simulink subsystem "PvtSubSys_HMI"  (R2020b)
settings: Solver=VariableStepAuto  StartTime=0.0  StopTime=10.0  RelTol=1e-3
undefined symbols (not defined in the file): P_HMI_LDW_LKAWarnTime, P_HMI_ObjectTypeFilter, P_HMI_WarnFormLDWReq
libraries: simulink x212, TrueDurationTime x6
(part 4 of 8)

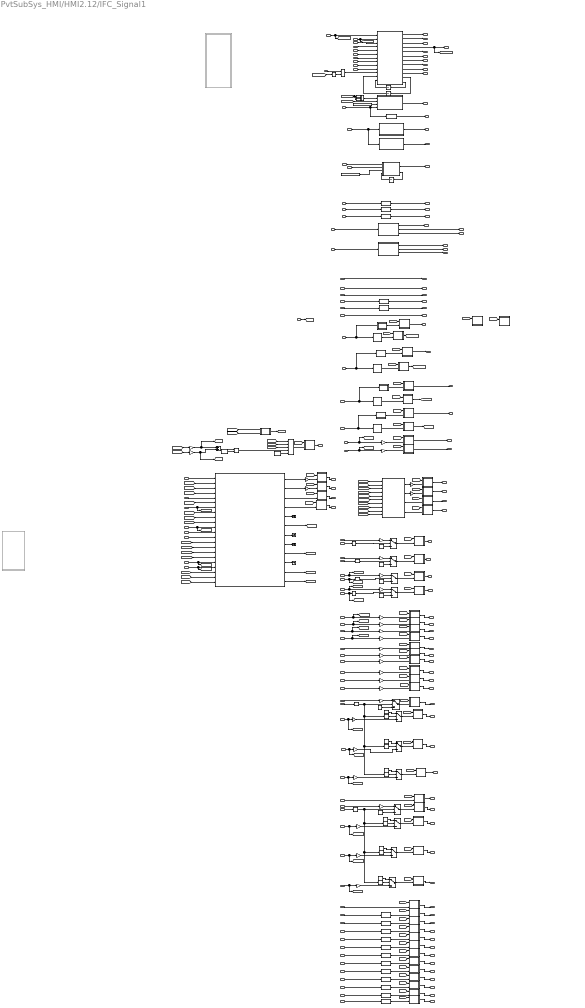
== system PvtSubSys_HMI/HMI2.12/IFC_Signal1 ==
  note: 按照开关请求
      | （ESS_PedSwtReq/ESS_VehSwtReq）
      | 进行正常值发送
  note: 需要添加 标定值
  note: 车道类型：目前只能显示车道线，还无法
      | 显示车道边界
  note: ELK 关联 3L功能 存在漏洞 2020/12/02
      |
      | 无故障：  0x0：No error
      | IFC故障： 0x2:LKA error
      | IFC无故障，RSDS故障：0x4:ELK error
      | error优先级：ELK>3L
      | （2）目前LKAResp 输出存在问题；无法与开关关联
      | 目前功能优先级；
      | TJA>ELK>3L
  note: 1.3.5——>1 solid
      | 2.4.6——>1 Dashed
      | 10.12.13——>1 Rode Edge
      | 8——>减速线（非虚线）
      | 14——>减速线（虚线）
  note: TJA_Off(0)
      |        TJA_Idle(1)
      |        TJA_Ready(2)
      |        TJA_Active(3)
      |        TJA_Error(7)
      |        TJA_SafeStop(9)
  note: Fusion:LaneAvailability
  note: Fusion:CameraBlockageSts
  note: Fusion:IFCCalibrationSts
  note: 0x0=UNDECIDED |
      | 0x1=SOLID |
      | 0x2=DASHED |
      | 0x3=DOUBLE_SOLID_DASHED |
      | 0x4=DOUBLE_DASHED_SOLID |
      | 0x5=DOUBLE_SOLID_SOLID |
      | 0x6=DOUBLE_DASHED_DASHED |
      | 0x7=BOTTS |
      | 0x8=DECELERATION |
      | 0x9=HOV_LANE |
      | 0xA=ROAD_EDGE |
      | 0xB=ELEVATED_STRUCTURE |
      | 0xC=LCURB |
      | 0xD=CONES_POLES |
      | 0xE=PARKED_CARS
  note: 0x0:Inactive
      | 0x1:Left Active
      | 0x2:Right active
      | 0x3:Reserved
  note: 0x0:Inactive
      | 0x1:Left Eva
      | 0x2:Right Eva
      | 0x3:Reserved
  note: 0x0:No intervention
      | 0x1:Left intervention
      | 0x2:Right intervention
      | 0x3:Reserved
  note: LSSIntervention：
      | 0x0:No warning and Intervention
      | 0x1: Left warning （报警voice ）
      | 0x2: Right warning
      | 0x3: Left Intervention
      | 0x4:Right Intervention
      | 0x5:Both Intervention (智慧躲闪/lck)
      | 0x6: Left warn only reminder(仅仅是提醒)
      | 0x7: Right warn only reminder
  note: 0x0:No display
      | 0x1:Solid lane
      | 0x2:Dashed lane
      | 0X3:Rode edge
      | 0X4-0x7:Reserved
  note: 0x0:ELK-OFF(关闭)
      | 0x1:ELK-Standby(开启)
      | 0x2:ELK-Enable(已使能，不满足扭矩介入条件)
      | 0x3:ELK-Road edge Active(道路边缘扭矩介入)
      | 0x4:ELK-Oncoming Active（oncoming扭矩介入）
      | 0x5:ELK-Overtaking Active（overtaking扭矩介入）
      | 0x6:ELK-Failure
      | 0x7:Reserved
  note: OFF(0)
      |         IDLE(1)
      |         READY(2)
      |         ACTIVE(3)
      |         ACTIVE_LEFT(4)
      |         ACTIVE_RIGHT(5)
      |         ERROR(6)
      |         DEFAULT(7)
  note: LSS haptic warning Request
  note: 0x0:Not Avaliable
      | 0x1:Left Lane Marker Available
      | 0x2:Right Lane Marker Available
      | 0x3:Both Lane Markers Available
  note: 0x0:No Request
      | 0x1:LeveL 1
      | 0x2~0x3:Reserved
  note: 0x0:Voice
      | 0x1:Haptic
      | 0x2:Voice+Haptic
      | 0x3:Reserved
  note: LDW(Lane Detection Warning)_LKA( Lane Keeping Assist) Sensitivity
  note: LSS_WarnFormSwtReq
  note: 0x0:Voice
      | 0x1:Haptic
      | 0x2:Voice+Haptic
      | 0x3:Reserved
  note: LSS Warning Form Switch status
  note: Fusion:IFCHUTInterface
  note: 0x0:Calibration Success
      | 0x1:Calibration In Process
      | 0x2:Calibration Failed
      | 0x3:Reserved
  note: 0x0:No intervention
      | 0x1:Left intervention
      | 0x2:Right intervention
      | 0x3:Reserved
  note: 0x0:undecided
      | 0x1:solid
      | 0x2:dashed
      | 0x3:double solid dashed
      | 0x4:double dashed solid
      | 0x5:double solid solid
      | 0x6:double dashed dashed
      | 0x7:botts
      | 0x8:deceleration
      | 0x9:hov_lane
      | 0xA:road edge
      | 0xB:elevated_structure
      | 0xC:curb
      | 0xD:cones_poles
  note: 本车道左侧车道线
  note: 本车道右侧车道线
  note: 左侧车道左侧车道线
  note: 右侧车道右侧车道线
  note: 0x0:OFF
      | 0x1:ON
      | 0x2-0x3:Reserved
  note: OFF = 0;
      | IDLE = 1;
      | READY = 2;
      | ACTIVE = 3;
      | ACTIVE_LEFT = 4;
      | ACTIVE_RIGHT = 5;
      | ERROR = 6;
  note: 红色Port为新加的信号
      |                                      ——2020/8/18
      |
      | (1)增加了ELK和LCK/LKA互动关系逻辑；
      | 修正LSSErrSts逻辑；
      | (2)增加了LSSSwt总开关逻辑；只有在LSSSwt打
      | 开的情况下，才能在3L功能任选其一；
      | (3)增加了LCKIESts信号；方便HUT开关逻辑编写；
      |                                      ——2020/11/03
      |
      | （1）LDW_LKAWarn该信号接地
      | （2）释放AES信号；
      |                                      ——2020/11/13
      |
      | （1） 增加了L1blsLineExist/ R1blsLineExist 两个信号；
      | 用来计算IFC_LaneCurve；
      | （2）关联TJAState与LSSIntervention；
      | （3）关联LSS_WarnFormSwtReq与LSSIntervention；
      | （4）增加LSSSwtReq 信号的“软开关”；修改横向功能
      | 输出；
      | （5）增加了LDW_LKAWarn信号输出
      | （6）增加了F_LBblsLineExist和F_RBblsLineExist两条
      | 边界有效性信号，用于输出计算仪表车道线信息；
      |                                       ——2020/11/30
      |
      | （1）IFCvibrationwarning信号关联LSSInTervention信号
      | only reminder coding值；
      | （2）关联TJAState与LSSIntervention及其横向状态；
      |
      |                                      ——2020/12/02
  note: 0x0:No LDW_LKA warning
      | 0x1:LDW_LKA left warning
      | 0x2:LDW_LKA right warning
      | 0x3:Reserved
  note: 0x0:No error
      | 0x1:LDW error
      | 0x2:LKA error
      | 0x3:LCK error
      | 0x4:ELK error
      | 0x5:ESS error
      | 0x6~0x7:Reserved
  note: 0x0:OFF
      | 0x1:ON
  note: 目前，还没有添加ESS
  note: 0x0:OFF
      | 0x1:LDW on
      | 0x2:LKA on
      | 0x3:LCK ON
      | 0x4~0x7:Reserved
  note: 0x0:No response
      | 0x1:Response
  note: 0x0=UNDECIDED
      | 0x1=SOLID
      | 0x2=DASHED
      | 0x3=DOUBLE_SOLID_DASHED
      | 0x4=DOUBLE_DASHED_SOLID
      | 0x5=DOUBLE_SOLID_SOLID
      | 0x6=DOUBLE_DASHED_DASHED
      | 0x7=BOTTS 路钉
      | 0x8=DECELERATION 减速线
      | 0x9=HOV_LANE 菱形线
      | 0xA=ROAD_EDGE
      | 0xB=ELEVATED_STRUCTURE
      | 0xC=LCURB
      | 0xD=CONES_POLES
      | 0xE=PARKED_CARS
      | 20:减速虚线
  note: 目前没有AES功能；
      | 20201031
  note: TJA_FollowSts
  note: ELK_OFF(0)
      |         ELK_IDLE(1)
      |         ELK_READY(2)
      |         ELK_ACTIVE_LEFT(3)
      |         ELK_ACTIVE_RIGHT(4)
      |         ELK_ONCOMING_LEFT(5)
      |         ELK_ONCOMING_RIGHT(6)
      |         ELK_OVERTAKING_LEFT(7)
      |         ELK_OVERTAKING_RIGHT(8)
      |         ELK_ERROR(9)
  note: 0x0:No Error
      | 0x1:Error
  note: 0x0:No display
      | 0x1:Solid lane
      | 0x2:Dashed lane
      | 0X3:Rode edge
      | 0X4-0x7:Reserved
  note: 仪表显示文档里的系数
  note: 0x0=UNDECIDED |
      | 0x1=SOLID |
      | 0x2=DASHED | 0x3=DOUBLE_SOLID_DASHED |
      | 0x4=DOUBLE_DASHED_SOLID |
      | 0x5=DOUBLE_SOLID_SOLID |
      | 0x6=DOUBLE_DASHED_DASHED |
      | 0x7=BOTTS |
      | 0x8=DECELERATION |
      | 0x9=HOV_LANE |
      | 0xA=ROAD_EDGE |
      | 0xB=ELEVATED_STRUCTURE |
      | 0xC=LCURB |
      | 0xD=CONES_POLES |
      | 0xE=PARKED_CARS |
      | 0xF=DLM_UNDECIDED |
      | 0x10=PHYSICAL_DIVIDER |
      | 0x11=FENCE |
      | 0x12=GUARDRAIL |
      | 0x13=WALL
  note: uint8
  note: single
  LSSSwtReq : Inport
  LDWState : Inport  Port=2
  LKAState : Inport  Port=3
  LCKState : Inport  Port=4
  ELKSts : Inport  Port=5
  LKAWarning : Inport  Port=6
  LCKIESts : Inport  Port=7
  TJAState : Inport  Port=8
  LSS_WarnFormSwtReq : Inport  Port=9
  ESS_PedSwtReq : Inport  Port=10
  ESS_VehSwtReq : Inport  Port=11
  AESSts : Inport  Port=12
  AESSwtReq : Inport  Port=13
  ESSSts : Inport  Port=14
  LaneAvailability : Inport  Port=15
  IFC_SnvtySet : Inport  Port=16
  IFCCalibrationSts : Inport  Port=17
  IFCHUTInterface : Inport  Port=18
  CameraBlockageSts : Inport  Port=19
  TJA_FollowSts : Inport  Port=20
  L1enLineType : Inport  Port=21
  R1enLineType : Inport  Port=22
  L2enLineType : Inport  Port=23
  R2enLineType : Inport  Port=24
  L1dC2V : Inport  Port=25
  R1dC2V : Inport  Port=26
  "L1blsLineExist " : Inport  Port=27
  L1dC0V : Inport  Port=28
  "R1blsLineExist " : Inport  Port=29
  R1dC0V : Inport  Port=30
  L2dC0V : Inport  Port=31
  R2dC0V : Inport  Port=32
  L1dC3V : Inport  Port=33
  L1dC1V : Inport  Port=34
  R1dC3V : Inport  Port=35
  R1dC1V : Inport  Port=36
  L2dC2V : Inport  Port=37
  L2dC3V : Inport  Port=38
  L2dC1V : Inport  Port=39
  R2dC2V : Inport  Port=40
  R2dC3V : Inport  Port=41
  R2dC1V : Inport  Port=42
  F_LBblsLineExist : Inport  Port=43
  F_LBdC0V : Inport  Port=44
  F_LBdC1V : Inport  Port=45
  F_LBdC2V : Inport  Port=46
  F_LBdC3V : Inport  Port=47
  F_LBenLineType : Inport  Port=48
  F_RBblsLineExist : Inport  Port=49
  F_RBdC0V : Inport  Port=50
  F_RBdC1V : Inport  Port=51
  F_RBdC2V : Inport  Port=52
  F_RBdC3V : Inport  Port=53
  F_RBenLineType : Inport  Port=54
  LKASwtReq : Inport  Port=55
  LCKSwtReq : Inport  Port=56
  L1dDisStart : Inport  Port=57
  L1dDisFront : Inport  Port=58
  R1dDisStart : Inport  Port=59
  R1dDisFront : Inport  Port=60
  L2dDisStart : Inport  Port=61
  L2dDisFront : Inport  Port=62
  R2dDisStart : Inport  Port=63
  R2dDisFront : Inport  Port=64
  E1dDisStart : Inport  Port=65
  E1dDisFront : Inport  Port=66
  E2dDisFront : Inport  Port=67
  E2dDisStart : Inport  Port=68
  L2LineExist : Inport  Port=69
  R2LineExist : Inport  Port=70
  standstill : Inport  Port=71
  Compare To Constant{,2..6} (6 alike) : simulink/Logic and Bit Operations/Compare To Constant  relop=>  const=1  OutDataTypeStr=boolean
  Compare To Constant1 : simulink/Logic and Bit Operations/Compare To Constant  relop=>  const=0  OutDataTypeStr=boolean
  Compare To Constant7 : simulink/Logic and Bit Operations/Compare To Constant  relop===  const=4  OutDataTypeStr=boolean
  Compare To Constant8 : simulink/Logic and Bit Operations/Compare To Constant  relop===  const=5  OutDataTypeStr=boolean
  Constant : Constant  Value=P_HMI_LDW_LKAWarnTime
  Constant1 : Constant  Value=single(0)
  Constant{6..7,10..13} (6 alike) : Constant  Value=0  OutDataTypeStr=single
  Constant14 : Constant  Value=P_HMI_WarnFormLDWReq
  Constant18 : Constant  Value=single(2)
  Constant2 : Constant  Value=-1.75  OutDataTypeStr=single
  Constant3 : Constant  Value=1.75  OutDataTypeStr=single
  Constant4 : Constant  Value=-5.25  OutDataTypeStr=single
  Constant5 : Constant  Value=5.25  OutDataTypeStr=single
  Constant8 : Constant  Value=-5.25  OutDataTypeStr=single
  Constant9 : Constant  Value=5.25  OutDataTypeStr=single
  Data Type Conversion : DataTypeConversion  OutDataTypeStr=boolean
  Data Type Conversion{1..4} (4 alike) : DataTypeConversion
  Data Type Conversion{5..16} (12 alike) : DataTypeConversion  OutDataTypeStr=single
  Data Type Conversion17 : DataTypeConversion  OutDataTypeStr=boolean
  Direct Lookup Table (n-D){,1,3..4} (4 alike) : LookupNDDirect  NumberOfTableDimensions=1  Table=[0 1 2 1 2 1 2 2 1 0 3 0 3 3 2 0 0 0 0 0 2]  TableDataTypeStr=uint8
  Divide2 : Product  Inputs=*/
  ELKSts1 : InportShadow  Port=5
  ELKSts3 : InportShadow  Port=5
  F_LBblsLineExist1 : InportShadow  Port=43
  F_LBdC0V1 : InportShadow  Port=44
  F_RBblsLineExist1 : InportShadow  Port=49
  F_RBdC0V1 : InportShadow  Port=50
  Gain{,1..3,5,7,10,13..15,18..19} (12 alike) : Gain  Gain=-1  OutDataTypeStr=single
  Gain{8,11,16,20,22..23} (6 alike) : Gain  Gain=-2  OutDataTypeStr=single
  Gain{4,6,9,12,17,21} (6 alike) : Gain  Gain=-6  OutDataTypeStr=single
  Gain25 : Gain  Gain=2  OutDataTypeStr=single
  Gain26 : Gain  Gain=2  OutDataTypeStr=single
  Gain{29..32} (4 alike) : Gain  Gain=-1
  L1blsLineExist 2 : InportShadow  Port=27
  L1dC0V1 : InportShadow  Port=28
  LKAState1 : InportShadow  Port=3
  LSS_WarnFormSwtReq1 : InportShadow  Port=9
  Logical Operator{,1..5} (6 alike) : Logic  Operator=NOT  Inputs=1  AllPortsSameDT=off  OutDataTypeStr=boolean
  Logical Operator6 : Logic  Operator=OR  AllPortsSameDT=off  OutDataTypeStr=boolean
  Logical Operator7 : Logic  AllPortsSameDT=off  OutDataTypeStr=boolean
  MATLAB Function : MATLAB Function  TreatAsAtomicUnit=on
  MATLAB Function1 : MATLAB Function  TreatAsAtomicUnit=on
  MATLAB Function10 : MATLAB Function  TreatAsAtomicUnit=on
  MATLAB Function11 : MATLAB Function  TreatAsAtomicUnit=on
  MATLAB Function12 : MATLAB Function  TreatAsAtomicUnit=on
  MATLAB Function13 : MATLAB Function  TreatAsAtomicUnit=on
  MATLAB Function2 : MATLAB Function  Commented=on  TreatAsAtomicUnit=on
  MATLAB Function3 : MATLAB Function  TreatAsAtomicUnit=on
  MATLAB Function4 : MATLAB Function  TreatAsAtomicUnit=on
  MATLAB Function5 : MATLAB Function  TreatAsAtomicUnit=on
  MATLAB Function7 : MATLAB Function  TreatAsAtomicUnit=on
  MATLAB Function8 : MATLAB Function  TreatAsAtomicUnit=on
  MATLAB Function9 : MATLAB Function  TreatAsAtomicUnit=on
  Multiport Switch : MultiPortSwitch  DataPortOrder=Specify indices  DataPortIndices={1,2,3,4}  DiagnosticForDefault=None
  R1blsLineExist 2 : InportShadow  Port=29
  R1dC0V1 : InportShadow  Port=30
  Subsystem : Subsystem
  Subsystem1 : Subsystem
  Subsystem10 : Subsystem
  Subsystem11 : Subsystem
  Subsystem12 : Subsystem
  Subsystem13 : Subsystem
  Subsystem14 : Subsystem
  Subsystem15 : Subsystem
  Subsystem16 : Subsystem
  Subsystem17 : Subsystem
  Subsystem18 : Subsystem
  Subsystem19 : Subsystem
  Subsystem2 : Subsystem  Commented=on
  Subsystem20 : Subsystem
  Subsystem21 : Subsystem
  Subsystem22 : Subsystem
  Subsystem23 : Subsystem
  Subsystem24 : Subsystem
  Subsystem25 : Subsystem
  Subsystem26 : Subsystem
  Subsystem27 : Subsystem
  Subsystem28 : Subsystem
  Subsystem29 : Subsystem
  Subsystem3 : Subsystem
  Subsystem30 : Subsystem
  Subsystem31 : Subsystem
  Subsystem32 : Subsystem
  Subsystem33 : Subsystem
  Subsystem34 : Subsystem
  Subsystem35 : Subsystem
  Subsystem36 : Subsystem
  Subsystem37 : Subsystem
  Subsystem38 : Subsystem
  Subsystem39 : Subsystem
  Subsystem4 : Subsystem
  Subsystem40 : Subsystem
  Subsystem41 : Subsystem
  Subsystem42 : Subsystem
  Subsystem43 : Subsystem
  Subsystem44 : Subsystem
  Subsystem45 : Subsystem
  Subsystem46 : Subsystem
  Subsystem47 : Subsystem
  Subsystem48 : Subsystem
  Subsystem49 : Subsystem
  Subsystem5 : Subsystem
  Subsystem50 : Subsystem
  Subsystem51 : Subsystem
  Subsystem52 : Subsystem
  Subsystem53 : Subsystem
  Subsystem54 : Subsystem
  Subsystem55 : Subsystem
  Subsystem56 : Subsystem
  Subsystem57 : Subsystem
  Subsystem58 : Subsystem
  Subsystem59 : Subsystem
  Subsystem6 : Subsystem
  Subsystem7 : Subsystem
  Subsystem8 : Subsystem
  Subsystem9 : Subsystem
  Subtract : Sum
  Switch{,1..4,6..7,9,14,17,20,23} (12 alike) : Switch  Criteria=u2 ~= 0
  Terminator{1..2,4,6} (4 alike) : Terminator
  Unit Delay : UnitDelay  SampleTime=-1  HasFrameUpgradeWarning=on
  Unit Delay1 : UnitDelay  InitialCondition=50  SampleTime=-1  HasFrameUpgradeWarning=on
  Unit Delay2 : UnitDelay  InitialCondition=50  SampleTime=-1  HasFrameUpgradeWarning=on
  LSSFuncSts : Outport
  LSSErrSts : Outport  Port=2
  LSSResp : Outport  Port=3
  LSSIntervention : Outport  Port=4
  LSSWarnFormResp : Outport  Port=5
  ELKResp : Outport  Port=6
  LCKResp : Outport  Port=7
  LKAResp : Outport  Port=8
  LDWResp : Outport  Port=9
  IntelligentEvaResp : Outport  Port=10
  IntelligentEvaActSts : Outport  Port=11
  ELKMainState : Outport  Port=12
  ELKActSts : Outport  Port=13
  LDW_LKAWarn : Outport  Port=14
  IFCVibrationWarning : Outport  Port=15
  ESS_PedResp : Outport  Port=16
  ESS_VehResp : Outport  Port=17
  AESResp : Outport  Port=18
  AESintervention : Outport  Port=19
  AES_Sts : Outport  Port=20
  AESErrSts : Outport  Port=21
  ESSintervention : Outport  Port=22
  ESS_Sts : Outport  Port=23
  ESSErrSts : Outport  Port=24
  IFC_LaneAvailability : Outport  Port=25
  LDW_LKA_Snvty : Outport  Port=26
  IFC_CalibrationSts : Outport  Port=27
  IFC_HUTInterface : Outport  Port=28
  Camera_BlockageSts : Outport  Port=29
  TJAFollowSts : Outport  Port=30
  IFC_LeLaneTyp : Outport  Port=31
  IFC_Line01_Type : Outport  Port=32
  IFC_RiLaneTyp : Outport  Port=33
  IFC_Line02_Type : Outport  Port=34
  IFC_NextLeLaneTyp : Outport  Port=35
  IFC_Line03_Type : Outport  Port=36
  IFC_NextRiLaneTyp : Outport  Port=37
  IFC_Line04_Type : Outport  Port=38
  IFC_Line01_Curv : Outport  Port=39
  IFC_LaneCurve : Outport  Port=40
  IFC_Line02_Curv : Outport  Port=41
  IFC_LeLane_dy : Outport  Port=42
  IFC_Line01_Dy : Outport  Port=43
  IFC_RiLane_dy : Outport  Port=44
  IFC_Line02_Dy : Outport  Port=45
  IFC_NextLeLane_dy : Outport  Port=46
  IFC_Line03_Dy : Outport  Port=47
  IFC_NextRiLane_dy : Outport  Port=48
  IFC_Line04_Dy : Outport  Port=49
  IFC_Line01_CurvChange : Outport  Port=50
  IFC_Line01_HeadingAngle : Outport  Port=51
  IFC_Line02_CurvChange : Outport  Port=52
  IFC_Line02_HeadingAngle : Outport  Port=53
  IFC_Line03_Curv : Outport  Port=54
  IFC_Line03_CurvChange : Outport  Port=55
  IFC_Line03_HeadingAngle : Outport  Port=56
  IFC_Line04_Curv : Outport  Port=57
  IFC_Line04_CurvChange : Outport  Port=58
  IFC_Line04_HeadingAngle : Outport  Port=59
  IFC_Roadedge01_Dy : Outport  Port=60
  IFC_Roadedge01_HeadingAngle : Outport  Port=61
  IFC_Roadedge01_Curv : Outport  Port=62
  IFC_Roadedge01_CurvChange : Outport  Port=63
  IFC_Roadedge01_Type : Outport  Port=64
  IFC_Roadedge02_Dy : Outport  Port=65
  IFC_Roadedge02_HeadingAngle : Outport  Port=66
  IFC_Roadedge02_Curv : Outport  Port=67
  IFC_Roadedge02_CurvChange : Outport  Port=68
  IFC_Roadedge02_Type : Outport  Port=69
  IFC_Line01_DxStart : Outport  Port=70
  IFC_Line01_DxEnd : Outport  Port=71
  IFC_Line02_DxStart : Outport  Port=72
  IFC_Line02_DxEnd : Outport  Port=73
  IFC_Line03_DxStart : Outport  Port=74
  IFC_Line03_DxEnd : Outport  Port=75
  IFC_Line04_DxStart : Outport  Port=76
  IFC_Line04_DxEnd : Outport  Port=77
  IFC_Roadedge01_DxStart : Outport  Port=78
  IFC_Roadedge01_DxEnd : Outport  Port=79
  IFC_Roadedge02_DxStart : Outport  Port=80
  IFC_Roadedge02_DxEnd : Outport  Port=81
  wires:
  Subsystem1/4(R1_Type) -> Subsystem57/2(in)
  [standstill] -> Subsystem57/1(standstill)
  Subsystem1/3(L1_Type) -> Subsystem56/2(in)
  [standstill] -> Subsystem56/1(standstill)
  Gain30/1 -> Subsystem55/2(in)
  [standstill] -> Subsystem55/1(standstill)
  Gain29/1 -> Subsystem54/2(in)
  [standstill] -> Subsystem54/1(standstill)
  Multiport Switch/1 -> Subsystem53/2(in)
  [standstill] -> Subsystem53/1(standstill)
  Switch23/1 -> Subsystem39/2(in)
  [standstill] -> Subsystem39/1(standstill)
  Switch20/1 -> Subsystem38/2(in)
  [standstill] -> Subsystem38/1(standstill)
  Switch17/1 -> Subsystem37/2(in)
  [standstill] -> Subsystem37/1(standstill)
  Switch7/1 -> Subsystem36/2(in)
  [standstill] -> Subsystem36/1(standstill)
  F_LBenLineType/1 -> Subsystem35/2(in)
  [standstill] -> Subsystem35/1(standstill)
  Subsystem35/1(out) -> IFC_Roadedge01_Type/1
  [standstill] -> Subsystem34/1(standstill)
  Switch9/1 -> Subsystem33/2(in)
  [standstill] -> Subsystem33/1(standstill)
  Switch4/1 -> Subsystem32/2(in)
  [standstill] -> Subsystem32/1(standstill)
  Switch6/1 -> Subsystem31/2(in)
  [standstill] -> Subsystem31/1(standstill)
  Gain13/1 -> Subsystem30/2(in)
  [standstill] -> Subsystem30/1(standstill)
  Gain12/1 -> Subsystem28/2(in)
  [standstill] -> Subsystem28/1(standstill)
  Gain11/1 -> Subsystem29/2(in)
  [standstill] -> Subsystem29/1(standstill)
  Gain10/1 -> Subsystem27/2(in)
  [standstill] -> Subsystem27/1(standstill)
  Gain9/1 -> Subsystem26/2(in)
  [standstill] -> Subsystem26/1(standstill)
  Gain8/1 -> Subsystem25/2(in)
  [standstill] -> Subsystem25/1(standstill)
  [standstill] -> Subsystem24/1(standstill)
  Gain7/1 -> Subsystem24/2(in)
  Gain6/1 -> Subsystem23/2(in)
  [standstill] -> Subsystem23/1(standstill)
  Gain5/1 -> Subsystem22/2(in)
  [standstill] -> Subsystem22/1(standstill)
  Gain4/1 -> Subsystem21/2(in)
  [standstill] -> Subsystem21/1(standstill)
  Switch3/1 -> Subsystem20/2(in)
  [standstill] -> Subsystem20/1(standstill)
  Switch2/1 -> Subsystem19/2(in)
  [standstill] -> Subsystem19/1(standstill)
  Switch1/1 -> Subsystem18/2(in)
  [standstill] -> Subsystem18/1(standstill)
  Switch/1 -> Subsystem17/2(in)
  [standstill] -> Subsystem17/1(standstill)
  Gain32/1 -> Subsystem16/2(in)
  [standstill] -> Subsystem16/1(standstill)
  Gain31/1 -> Subsystem15/2(in)
  [standstill] -> Subsystem15/1(standstill)
  [standstill] -> Subsystem14/1(standstill)
  Subsystem/4(R2_Type) -> Subsystem14/2(in)
  Subsystem/3(L2_Type) -> Subsystem13/2(in)
  [standstill] -> Subsystem13/1(standstill)
  Gain22/1 -> Subsystem12/2(in)
  [standstill] -> Subsystem12/1(standstill)
  Gain23/1 -> Subsystem11/2(in)
  [standstill] -> Subsystem11/1(standstill)
  Direct Lookup Table (n-D)1/1 -> Subsystem10/2(in)
  [standstill] -> Subsystem10/1(standstill)
  MATLAB Function5/1(Type) -> Subsystem9/2(in)
  [standstill] -> Subsystem9/1(standstill)
  Direct Lookup Table (n-D)4/1 -> Subsystem8/2(in)
  [standstill] -> Subsystem8/1(standstill)
  MATLAB Function4/1(Type) -> Subsystem7/2(in)
  [standstill] -> Subsystem7/1(standstill)
  [standstill] -> Subsystem6/1(standstill)
  [standstill] -> Subsystem5/1(standstill)
  Direct Lookup Table (n-D)/1 -> Subsystem4/2(in)
  [standstill] -> Subsystem4/1(standstill)
  MATLAB Function1/1(Type) -> Subsystem3/2(in)
  [standstill] -> Subsystem3/1(standstill)
  [standstill] -> Subsystem59/1(standstill)
  ? -> Subsystem59/2(in)
  [standstill] -> Subsystem58/1(standstill)
  ? -> Subsystem58/2(in)
  Subsystem12/1(out) -> IFC_Line02_Curv/1
  Subsystem11/1(out) -> IFC_Line01_Curv/1
  Subsystem3/1(out) -> IFC_Line01_Type/1
  Subsystem5/1(out) -> IFC_Line02_Type/1
  Subsystem7/1(out) -> IFC_Line03_Type/1
  Subsystem9/1(out) -> IFC_Line04_Type/1
  Subsystem53/1(out) -> IFC_LaneCurve/1
  Subsystem57/1(out) -> IFC_RiLaneTyp/1
  Subsystem56/1(out) -> IFC_LeLaneTyp/1
  Subsystem55/1(out) -> IFC_RiLane_dy/1
  Subsystem54/1(out) -> IFC_LeLane_dy/1
  Subsystem15/1(out) -> IFC_NextLeLane_dy/1
  Subsystem16/1(out) -> IFC_NextRiLane_dy/1
  Subsystem13/1(out) -> IFC_NextLeLaneTyp/1
  Subsystem14/1(out) -> IFC_NextRiLaneTyp/1
  Subsystem52/1(out) -> IFC_Roadedge02_DxEnd/1
  Data Type Conversion16/1 -> Subsystem52/2(in)  "IFC_Roadedge02_DxEnd"
  [standstill] -> Subsystem52/1(standstill)
  Subsystem51/1(out) -> IFC_Roadedge02_DxStart/1
  Data Type Conversion11/1 -> Subsystem51/2(in)  "IFC_Roadedge02_DxStart"
  [standstill] -> Subsystem51/1(standstill)
  Subsystem50/1(out) -> IFC_Roadedge01_DxEnd/1
  Data Type Conversion14/1 -> Subsystem50/2(in)  "IFC_Roadedge01_DxEnd"
  [standstill] -> Subsystem50/1(standstill)
  Subsystem49/1(out) -> IFC_Roadedge01_DxStart/1
  Data Type Conversion15/1 -> Subsystem49/2(in)  "IFC_Roadedge01_DxStart"
  [standstill] -> Subsystem49/1(standstill)
  Subsystem48/1(out) -> IFC_Line04_DxEnd/1
  Data Type Conversion12/1 -> Subsystem48/2(in)  "IFC_Line04_DxEnd"
  [standstill] -> Subsystem48/1(standstill)
  Subsystem47/1(out) -> IFC_Line04_DxStart/1
  Data Type Conversion13/1 -> Subsystem47/2(in)  "IFC_Line04_DxStart"
  [standstill] -> Subsystem47/1(standstill)
  Subsystem46/1(out) -> IFC_Line03_DxEnd/1
  Data Type Conversion9/1 -> Subsystem46/2(in)  "IFC_Line03_DxEnd"
  [standstill] -> Subsystem46/1(standstill)
  Subsystem45/1(out) -> IFC_Line03_DxStart/1
  Data Type Conversion10/1 -> Subsystem45/2(in)  "IFC_Line03_DxStart"
  [standstill] -> Subsystem45/1(standstill)
  Subsystem44/1(out) -> IFC_Line02_DxEnd/1
  Data Type Conversion7/1 -> Subsystem44/2(in)  "IFC_Line02_DxEnd"
  [standstill] -> Subsystem44/1(standstill)
  Data Type Conversion8/1 -> Subsystem43/2(in)  "IFC_Line02_DxStart"
  Subsystem43/1(out) -> IFC_Line02_DxStart/1
  [standstill] -> Subsystem43/1(standstill)
  [standstill] -> Subsystem42/1(standstill)
  Subsystem42/1(out) -> IFC_Line01_DxEnd/1
  Data Type Conversion5/1 -> Subsystem42/2(in)  "IFC_Line01_DxEnd"
  [standstill] -> Subsystem41/1(standstill)
  Data Type Conversion6/1 -> Subsystem41/2(in)  "IFC_Line01_DxStart"
  Subsystem41/1(out) -> IFC_Line01_DxStart/1
  Subsystem40/1(out) -> IFC_Roadedge02_Type/1
  F_RBenLineType/1 -> Subsystem40/2(in)
  [standstill] -> Subsystem40/1(standstill)
  Subsystem39/1(out) -> IFC_Roadedge02_CurvChange/1
  Subsystem38/1(out) -> IFC_Roadedge02_HeadingAngle/1
  Subsystem37/1(out) -> IFC_Roadedge02_Curv/1
  Subsystem36/1(out) -> IFC_Roadedge02_Dy/1
  Subsystem34/1(out) -> IFC_Roadedge01_CurvChange/1
  Switch14/1 -> Subsystem34/2(in)
  Subsystem33/1(out) -> IFC_Roadedge01_HeadingAngle/1
  Subsystem32/1(out) -> IFC_Roadedge01_Curv/1
  Subsystem31/1(out) -> IFC_Roadedge01_Dy/1
  Subsystem30/1(out) -> IFC_Line04_HeadingAngle/1
  Subsystem28/1(out) -> IFC_Line04_CurvChange/1
  Subsystem29/1(out) -> IFC_Line04_Curv/1
  Subsystem27/1(out) -> IFC_Line03_HeadingAngle/1
  Subsystem26/1(out) -> IFC_Line03_CurvChange/1
  Subsystem25/1(out) -> IFC_Line03_Curv/1
  Subsystem24/1(out) -> IFC_Line02_HeadingAngle/1
  Subsystem23/1(out) -> IFC_Line02_CurvChange/1
  Subsystem22/1(out) -> IFC_Line01_HeadingAngle/1
  Subsystem21/1(out) -> IFC_Line01_CurvChange/1
  Subsystem20/1(out) -> IFC_Line04_Dy/1
  Subsystem19/1(out) -> IFC_Line03_Dy/1
  Subsystem18/1(out) -> IFC_Line02_Dy/1
  Subsystem17/1(out) -> IFC_Line01_Dy/1
  Subsystem10/1(out) -> [R2enLineType]
  Subsystem8/1(out) -> [L2enLineType]
  Subsystem6/1(out) -> [Lane_RiLaneTyp]
  Direct Lookup Table (n-D)3/1 -> Subsystem6/2(in)
  MATLAB Function13/1(Type) -> Subsystem5/2(in)
  Subsystem4/1(out) -> [Lane_LeLaneTyp]
  standstill/1 -> [standstill]
  Unit Delay2/1 -> MATLAB Function3/13(Rcountk1)
  MATLAB Function3/12(Rcount) -> Unit Delay2/1
  Unit Delay1/1 -> MATLAB Function3/12(Lcountk1)
  MATLAB Function3/11(Lcount) -> Unit Delay1/1
  Data Type Conversion17/1 -> Camera_BlockageSts/1
  MATLAB Function12/1(ELKActSts) -> ELKActSts/1
  MATLAB Function3/10(IntelligentEvaActSts) -> IntelligentEvaActSts/1
  [L2dC0V] -> Subsystem/1(L2_A0)
  [R2dC0V] -> Subsystem/2(R2_A0)
  [R2LineExist] -> Subsystem/7(R2Valid)
  [L2LineExist] -> Subsystem/5(L2Valid)
  [R2enLineType] -> Subsystem/10(Right_type)
  [L2enLineType] -> Subsystem/9(Left_type)
  [F_LBdC0V] -> Subsystem/3(LReA0)
  [F_RBdC0V] -> Subsystem/4(RReA0)
  [F_RBblsLineExist] -> Subsystem/8(RReValid)
  [F_LBblsLineExist] -> Subsystem/6(LReValid)
  Subsystem/2(R2_ValidLaneA0) -> Gain32/1
  Subsystem/1(L2_ValidLaneA0) -> Gain31/1
  Subsystem1/5(L1_A1) -> Terminator6/1
  Subsystem1/7(L1_A3) -> Terminator4/1
  Subsystem1/8(R1_A1) -> Terminator2/1
  Subsystem1/10(R1_A3) -> Terminator1/1
  Gain26/1 -> Subtract/2, [Ri_Curv]
  Gain25/1 -> Subtract/1, [Le_Curv]
  [R1_A2] -> Gain26/1
  [L1_A2] -> Gain25/1
  Subsystem1/12(R1_Valid1) -> [R_Valid]
  Subsystem1/11(L1_Valid) -> [L_Valid]
  R1dC2V/1 -> Gain22/1, [R1dC2V]
  L1dC2V/1 -> Gain23/1, [L1dC2V]
  Subsystem1/9(R1_A2) -> [R1_A2]
  Subsystem1/6(L1_A2) -> [L1_A2]
  [RbdC1V] -> Subsystem1/20(Right_ReA1)
  [RbdC2V] -> Subsystem1/21(Right_ReA2)
  [RbdC3V] -> Subsystem1/22(Right_ReA3)
  F_RBdC1V/1 -> Gain18/1, [RbdC1V]
  F_RBdC2V/1 -> Gain20/1, [RbdC2V]
  [LbdC3V] -> Subsystem1/10(Left_ReA3)
  [LbdC1V] -> Subsystem1/8(Left_ReA1)
  F_LBdC1V/1 -> Gain15/1, [LbdC1V]
  [LbdC2V] -> Subsystem1/9(Left_ReA2)
  [R1dC2V] -> Subsystem1/15(Right_LaneA2)
  [L1dC2V] -> Subsystem1/3(Left_LaneA2)
  [L1dC3V] -> Subsystem1/4(Left_LaneA3)
  [R1dC3V] -> Subsystem1/16(Right_LaneA3)
  [R1dC1V] -> Subsystem1/14(Right_LaneA1)
  [L1dC1V] -> Subsystem1/2(Left_LaneA1)
  Compare To Constant3/1 -> Switch2/2
  Constant14/1 -> MATLAB Function8/3(warnform)
  Logical Operator6/1 -> MATLAB Function8/1(LDWActive)
  Compare To Constant8/1 -> Logical Operator6/1
  Compare To Constant7/1 -> Logical Operator6/2
  [LDWState] -> Compare To Constant8/1, Compare To Constant7/1
  Gain21/1 -> Switch23/3
  F_RBblsLineExist1/1 -> Compare To Constant6/1
  Logical Operator5/1 -> Switch23/2
  Constant13/1 -> Switch23/1
  Constant12/1 -> Switch20/1
  Logical Operator4/1 -> Switch20/2
  Gain18/1 -> Switch20/3
  Gain20/1 -> Switch17/3
  Logical Operator3/1 -> Switch17/2
  Constant11/1 -> Switch17/1
  Constant10/1 -> Switch14/1
  Logical Operator2/1 -> Switch14/2
  F_LBblsLineExist1/1 -> Compare To Constant5/1
  Gain17/1 -> Switch14/3
  Gain15/1 -> Switch9/3
  Logical Operator1/1 -> Switch9/2
  Constant7/1 -> Switch9/1
  Constant6/1 -> Switch4/1
  Logical Operator/1 -> Switch4/2
  L2LineExist/1 -> Compare To Constant3/1, [L2LineExist]
  Constant9/1 -> Switch7/3
  Gain19/1 -> Switch7/1
  Constant8/1 -> Switch6/3
  Gain14/1 -> Switch6/1
  Constant5/1 -> Switch3/3
  R2LineExist/1 -> Compare To Constant4/1, [R2LineExist]
  Gain3/1 -> Switch3/1
  Constant4/1 -> Switch2/3
  Gain2/1 -> Switch2/1
  R1blsLineExist 2/1 -> Compare To Constant2/1
  Constant3/1 -> Switch1/3
  Gain1/1 -> Switch1/1
  Constant2/1 -> Switch/3
  Gain/1 -> Switch/1
  L1blsLineExist 2/1 -> Compare To Constant/1
  E2dDisFront/1 -> Data Type Conversion16/1
  E2dDisStart/1 -> Data Type Conversion11/1
  E1dDisFront/1 -> Data Type Conversion14/1
  E1dDisStart/1 -> Data Type Conversion15/1
  R2dDisFront/1 -> Data Type Conversion12/1
  R2dDisStart/1 -> Data Type Conversion13/1
  L2dDisFront/1 -> Data Type Conversion9/1
  L2dDisStart/1 -> Data Type Conversion10/1
  R1dDisFront/1 -> Data Type Conversion7/1
  R1dDisStart/1 -> Data Type Conversion8/1
  L1dDisFront/1 -> Data Type Conversion5/1
  L1dDisStart/1 -> Data Type Conversion6/1
  [LSSIntervention] -> MATLAB Function8/2(LSSIntervention)
  Divide2/1 -> Multiport Switch/4
  Gain16/1 -> Switch4/3
  LCKIESts/1 -> MATLAB Function3/7(LCKIESts)
  Data Type Conversion/1 -> IFC_HUTInterface/1
  IFC_SnvtySet/1 -> LDW_LKA_Snvty/1
  MATLAB Function3/9(IntelligentEvaResp) -> IntelligentEvaResp/1
  MATLAB Function3/8(LDWResp) -> LDWResp/1
  MATLAB Function3/7(LKAResp) -> LKAResp/1
  MATLAB Function3/6(LCKResp) -> LCKResp/1
  MATLAB Function3/5(ELKResp) -> ELKResp/1
  MATLAB Function3/4(LSSIntervention) -> LSSIntervention/1, [LSSIntervention]
  LKAWarning/1 -> MATLAB Function3/6(LKAWarning)
  Data Type Conversion1/1 -> LSSWarnFormResp/1
  MATLAB Function7/3(Error) -> ESSErrSts/1
  MATLAB Function7/2(State) -> ESS_Sts/1
  MATLAB Function9/3(Error) -> AESErrSts/1
  MATLAB Function9/2(State) -> AES_Sts/1
  AESSts/1 -> MATLAB Function9/1(ESSSts)
  F_RBdC3V/1 -> Gain21/1, [RbdC3V]
  F_RBdC0V/1 -> Gain19/1
  F_LBdC3V/1 -> Gain17/1, [LbdC3V]
  F_LBdC2V/1 -> Gain16/1, [LbdC2V]
  F_LBdC0V/1 -> Gain14/1
  R2dC1V/1 -> Gain13/1
  L2dC1V/1 -> Gain10/1
  R1dC1V/1 -> Gain7/1, [R1dC1V]
  L1dC1V/1 -> Gain5/1, [L1dC1V]
  R2dC3V/1 -> Gain12/1
  R2dC2V/1 -> Gain11/1
  L2dC3V/1 -> Gain9/1
  L2dC2V/1 -> Gain8/1
  R1dC3V/1 -> Gain6/1, [R1dC3V]
  L1dC3V/1 -> Gain4/1, [L1dC3V]
  ESSSts/1 -> MATLAB Function7/1(ESSSts)
  MATLAB Function7/1(Intervention) -> ESSintervention/1
  MATLAB Function9/1(Intervention) -> AESintervention/1
  MATLAB Function3/1(LSSFuncSts) -> LSSFuncSts/1
  MATLAB Function3/2(LSSErrSts) -> LSSErrSts/1
  MATLAB Function3/3(LSSResp) -> LSSResp/1
  ELKSts/1 -> MATLAB Function3/5(ELKSts)
  LCKState/1 -> MATLAB Function3/4(LCKState)
  LKAState/1 -> MATLAB Function3/3(LKAState)
  LDWState/1 -> [LDWState], MATLAB Function3/2(LDWState)
  CameraBlockageSts/1 -> Data Type Conversion17/1
  IFCHUTInterface/1 -> Data Type Conversion/1
  IFCCalibrationSts/1 -> IFC_CalibrationSts/1
  AESSwtReq/1 -> Data Type Conversion4/1
  ESS_VehSwtReq/1 -> Data Type Conversion3/1
  ESS_PedSwtReq/1 -> Data Type Conversion2/1
  LSS_WarnFormSwtReq1/1 -> MATLAB Function8/4(WarnFormReq), Data Type Conversion1/1
  LSS_WarnFormSwtReq/1 -> MATLAB Function3/9(LSS_WarnFormSwtReq)
  TJA_FollowSts/1 -> TJAFollowSts/1
  LaneAvailability/1 -> IFC_LaneAvailability/1
  MATLAB Function8/1(y) -> IFCVibrationWarning/1
  MATLAB Function/1(ELKmainState) -> ELKMainState/1
  ELKSts3/1 -> MATLAB Function/1(ELKState), MATLAB Function12/1(ELKState)
  TJAState/1 -> MATLAB Function3/8(TJAState)
  R2dC0V/1 -> Gain3/1, [R2dC0V]
  L2dC0V/1 -> Gain2/1, [L2dC0V]
  R1dC0V/1 -> Gain1/1
  L1dC0V/1 -> Gain/1
  Constant18/1 -> Divide2/2
  Subtract/1 -> Divide2/1
  R2enLineType/1 -> MATLAB Function5/1(fType), Direct Lookup Table (n-D)1/1
  L2enLineType/1 -> MATLAB Function4/1(fType), Direct Lookup Table (n-D)4/1
  R1enLineType/1 -> MATLAB Function13/1(fType), Direct Lookup Table (n-D)3/1
  L1enLineType/1 -> Direct Lookup Table (n-D)/1, MATLAB Function1/1(fType)
  LSSSwtReq/1 -> [LSSSwtReq], MATLAB Function3/1(LSSSwtReq)
  MATLAB Function11/1(LDW_LKAWarn) -> LDW_LKAWarn/1
  Data Type Conversion2/1 -> ESS_PedResp/1
  Data Type Conversion3/1 -> ESS_VehResp/1
  Data Type Conversion4/1 -> AESResp/1
  [L_Valid] -> MATLAB Function10/1(Lvalid)
  [R_Valid] -> MATLAB Function10/2(Rvalid)
  MATLAB Function10/1(y) -> [SelectLane]
  [SelectLane] -> Multiport Switch/1
  Constant1/1 -> Multiport Switch/5
  [Le_Curv] -> Multiport Switch/2
  [Ri_Curv] -> Multiport Switch/3
  MATLAB Function11/2(count) -> Unit Delay/1
  Unit Delay/1 -> MATLAB Function11/4(countk1)
  LKAState1/1 -> MATLAB Function11/2(LKAState)
  ELKSts1/1 -> MATLAB Function11/1(ELKSts)
  L1dC0V1/1 -> Subsystem1/1(Left_LaneA0)
  R1dC0V1/1 -> Subsystem1/13(Right_LaneA0)
  F_LBdC0V1/1 -> Subsystem1/7(Left_ReA0), [F_LBdC0V]
  F_RBdC0V1/1 -> Subsystem1/19(Right_ReA0), [F_RBdC0V]
  "L1blsLineExist "/1 -> Subsystem1/5(Left_LaneValid)
  "R1blsLineExist "/1 -> Subsystem1/12(Right_LaneValid)
  F_LBblsLineExist/1 -> Subsystem1/11(Left_ReValid), [F_LBblsLineExist]
  F_RBblsLineExist/1 -> Subsystem1/18(Right_ReValid), [F_RBblsLineExist]
  Subsystem1/1(L1_A0) -> Gain29/1
  Subsystem1/2(Right_A0) -> Gain30/1
  Constant/1 -> MATLAB Function11/3(Time)
  [Lane_LeLaneTyp] -> Subsystem1/6(L1_type)
  [Lane_RiLaneTyp] -> Subsystem1/17(Right_type)
  LKASwtReq/1 -> MATLAB Function3/10(LKASwtReq)
  [LSSSwtReq] -> Compare To Constant1/1
  Compare To Constant1/1 -> Logical Operator7/2
  Logical Operator7/1 -> MATLAB Function3/11(LCKSwtReq)
  LCKSwtReq/1 -> Logical Operator7/1
  Compare To Constant/1 -> Switch/2
  Compare To Constant2/1 -> Switch1/2
  Compare To Constant4/1 -> Switch3/2
  Compare To Constant5/1 -> Switch6/2, Logical Operator1/1, Logical Operator2/1, Logical Operator/1
  Compare To Constant6/1 -> Switch7/2, Logical Operator3/1, Logical Operator4/1, Logical Operator5/1

== system PvtSubSys_HMI/HMI2.12/HWA//ACC//TJA_Signal1/100ms1 ==
  In1 : Inport
  Logical Operator : Logic  Operator=OR  Inputs=5  AllPortsSameDT=off  OutDataTypeStr=boolean
  Unit Delay{1..4} (4 alike) : UnitDelay  SampleTime=-1  HasFrameUpgradeWarning=on
  Out1 : Outport
  wires:
  In1/1 -> Unit Delay1/1, Logical Operator/1
  Unit Delay1/1 -> Logical Operator/2, Unit Delay2/1
  Unit Delay2/1 -> Unit Delay3/1, Logical Operator/3
  Unit Delay3/1 -> Unit Delay4/1, Logical Operator/4
  Unit Delay4/1 -> Logical Operator/5
  Logical Operator/1 -> Out1/1

== system PvtSubSys_HMI/HMI2.12/HWA//ACC//TJA_Signal1/100ms2 ==
  In1 : Inport
  Logical Operator : Logic  Operator=OR  Inputs=5  AllPortsSameDT=off  OutDataTypeStr=boolean
  Unit Delay{1..4} (4 alike) : UnitDelay  SampleTime=-1  HasFrameUpgradeWarning=on
  Out1 : Outport
  wires:
  Logical Operator/1 -> Out1/1
  Unit Delay4/1 -> Logical Operator/5
  Unit Delay3/1 -> Logical Operator/4, Unit Delay4/1
  Unit Delay2/1 -> Logical Operator/3, Unit Delay3/1
  Unit Delay1/1 -> Unit Delay2/1, Logical Operator/2
  In1/1 -> Logical Operator/1, Unit Delay1/1

== system PvtSubSys_HMI/HMI2.12/HWA//ACC//TJA_Signal1/100ms3 ==
  In1 : Inport
  Logical Operator : Logic  Operator=OR  Inputs=5  AllPortsSameDT=off  OutDataTypeStr=boolean
  Unit Delay{1..4} (4 alike) : UnitDelay  SampleTime=-1  HasFrameUpgradeWarning=on
  Out1 : Outport
  wires:
  In1/1 -> Unit Delay1/1, Logical Operator/1
  Unit Delay1/1 -> Logical Operator/2, Unit Delay2/1
  Unit Delay2/1 -> Unit Delay3/1, Logical Operator/3
  Unit Delay3/1 -> Unit Delay4/1, Logical Operator/4
  Unit Delay4/1 -> Logical Operator/5
  Logical Operator/1 -> Out1/1

== system PvtSubSys_HMI/HMI2.12/HWA//ACC//TJA_Signal1/100ms4 ==
  In1 : Inport
  Logical Operator : Logic  Operator=OR  Inputs=5  AllPortsSameDT=off  OutDataTypeStr=boolean
  Unit Delay{1..4} (4 alike) : UnitDelay  SampleTime=-1  HasFrameUpgradeWarning=on
  Out1 : Outport
  wires:
  Logical Operator/1 -> Out1/1
  Unit Delay4/1 -> Logical Operator/5
  Unit Delay3/1 -> Logical Operator/4, Unit Delay4/1
  Unit Delay2/1 -> Logical Operator/3, Unit Delay3/1
  Unit Delay1/1 -> Unit Delay2/1, Logical Operator/2
  In1/1 -> Logical Operator/1, Unit Delay1/1

== system PvtSubSys_HMI/HMI2.12/HWA//ACC//TJA_Signal1/Enlong3s ==
  In1 : Inport
  Compare To Constant : simulink/Logic and Bit Operations/Compare To Constant  relop=>  const=0.5  OutDataTypeStr=boolean
  Detect Increase3 : simulink/Logic and Bit Operations/Detect Increase  vinit=0.0  OutDataTypeStr=boolean
  MATLAB Function : MATLAB Function  TreatAsAtomicUnit=on
  Switch20 : Switch  Criteria=u2 ~= 0
  Time : Constant  Value=3000/20  OutDataTypeStr=uint16
  Unit Delay : UnitDelay  SampleTime=-1  HasFrameUpgradeWarning=on
  Unit Delay2 : UnitDelay  SampleTime=-1  HasFrameUpgradeWarning=on
  Unit Delay3 : UnitDelay  SampleTime=-1  HasFrameUpgradeWarning=on
  Out1 : Outport
  wires:
  Detect Increase3/1 -> Unit Delay3/1
  Time/1 -> MATLAB Function/3(Num)
  Switch20/1 -> Out1/1, Unit Delay2/1
  Unit Delay2/1 -> Switch20/1
  Unit Delay3/1 -> MATLAB Function/2(X)
  Compare To Constant/1 -> Switch20/2
  MATLAB Function/1(Cnt) -> Compare To Constant/1, Unit Delay/1
  Unit Delay/1 -> MATLAB Function/1(CntK1)
  In1/1 -> Switch20/3, Detect Increase3/1

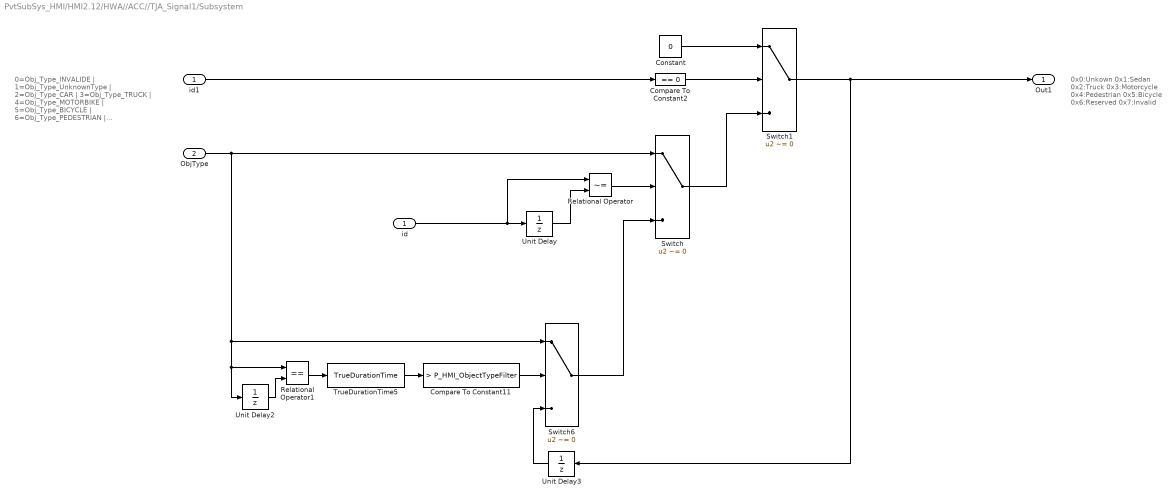
== system PvtSubSys_HMI/HMI2.12/HWA//ACC//TJA_Signal1/Subsystem ==
  note: 0x0:Unkown
      | 0x1:Sedan
      | 0x2:Truck
      | 0x3:Motorcycle
      | 0x4:Pedestrian
      | 0x5:Bicycle
      | 0x6:Reserved
      | 0x7:Invalid
  note: 0=Obj_Type_INVALIDE |
      | 1=Obj_Type_UnknownType |
      | 2=Obj_Type_CAR |
      | 3=Obj_Type_TRUCK |
      | 4=Obj_Type_MOTORBIKE |
      | 5=Obj_Type_BICYCLE |
      | 6=Obj_Type_PEDESTRIAN |
      | 7=Obj_Type_GENERAL_OBJECT |
      | 8=Obj_Type_ANIMAL|
  id : Inport
  ObjType : Inport  Port=2
  Compare To Constant11 : simulink/Logic and Bit Operations/Compare To Constant  relop=>  const=P_HMI_ObjectTypeFilter  OutDataTypeStr=boolean
  Compare To Constant2 : simulink/Logic and Bit Operations/Compare To Constant  relop===  const=0  OutDataTypeStr=boolean
  Constant : Constant  Value=0  OutDataTypeStr=uint8
  Relational Operator : RelationalOperator  Operator=~=  OutDataTypeStr=boolean  RndMeth=Simplest
  Relational Operator1 : RelationalOperator  Operator===  OutDataTypeStr=boolean  RndMeth=Simplest
  Switch : Switch  Criteria=u2 ~= 0
  Switch1 : Switch  Criteria=u2 ~= 0
  Switch6 : Switch  Criteria=u2 ~= 0
  TrueDurationTime5 : TrueDurationTime/TrueDurationTime  TCycle=0.02
  Unit Delay : UnitDelay  SampleTime=-1  HasFrameUpgradeWarning=on
  Unit Delay2 : UnitDelay  SampleTime=-1  HasFrameUpgradeWarning=on
  Unit Delay3 : UnitDelay  SampleTime=-1  HasFrameUpgradeWarning=on
  id1 : InportShadow
  Out1 : Outport
  wires:
  Relational Operator/1 -> Switch/2
  Switch/1 -> Switch1/3
  Compare To Constant2/1 -> Switch1/2
  id1/1 -> Compare To Constant2/1
  Constant/1 -> Switch1/1
  Unit Delay3/1 -> Switch6/3
  Compare To Constant11/1 -> Switch6/2
  Relational Operator1/1 -> TrueDurationTime5/1
  Unit Delay2/1 -> Relational Operator1/2
  TrueDurationTime5/1 -> Compare To Constant11/1
  Switch6/1 -> Switch/3
  ObjType/1 -> Switch6/1, Relational Operator1/1, Unit Delay2/1, Switch/1
  Switch1/1 -> Out1/1, Unit Delay3/1
  id/1 -> Unit Delay/1, Relational Operator/1
  Unit Delay/1 -> Relational Operator/2

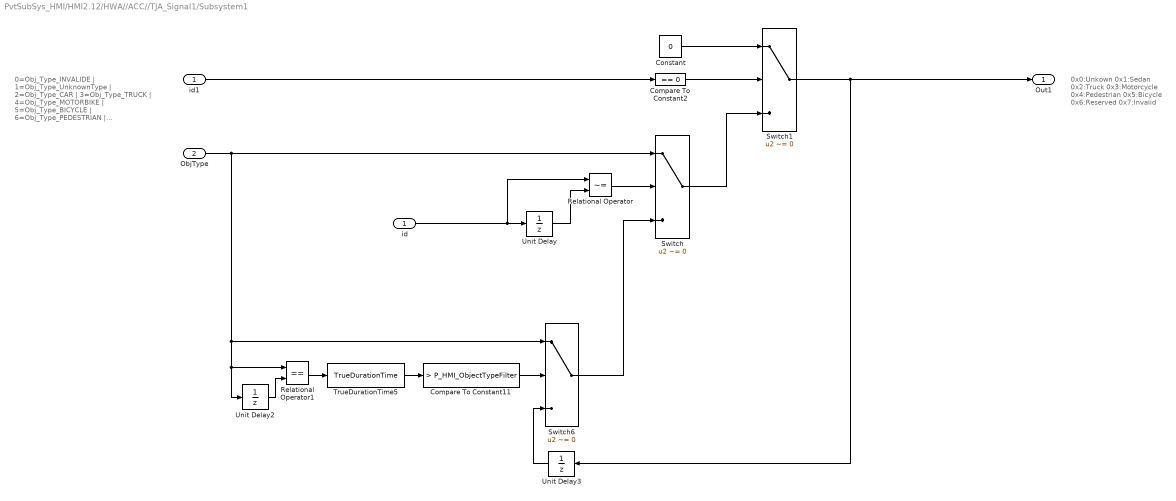
== system PvtSubSys_HMI/HMI2.12/HWA//ACC//TJA_Signal1/Subsystem1 ==
  note: 0=Obj_Type_INVALIDE |
      | 1=Obj_Type_UnknownType |
      | 2=Obj_Type_CAR |
      | 3=Obj_Type_TRUCK |
      | 4=Obj_Type_MOTORBIKE |
      | 5=Obj_Type_BICYCLE |
      | 6=Obj_Type_PEDESTRIAN |
      | 7=Obj_Type_GENERAL_OBJECT |
      | 8=Obj_Type_ANIMAL|
  note: 0x0:Unkown
      | 0x1:Sedan
      | 0x2:Truck
      | 0x3:Motorcycle
      | 0x4:Pedestrian
      | 0x5:Bicycle
      | 0x6:Reserved
      | 0x7:Invalid
  id : Inport
  ObjType : Inport  Port=2
  Compare To Constant11 : simulink/Logic and Bit Operations/Compare To Constant  relop=>  const=P_HMI_ObjectTypeFilter  OutDataTypeStr=boolean
  Compare To Constant2 : simulink/Logic and Bit Operations/Compare To Constant  relop===  const=0  OutDataTypeStr=boolean
  Constant : Constant  Value=0  OutDataTypeStr=uint8
  Relational Operator : RelationalOperator  Operator=~=  OutDataTypeStr=boolean  RndMeth=Simplest
  Relational Operator1 : RelationalOperator  Operator===  OutDataTypeStr=boolean  RndMeth=Simplest
  Switch : Switch  Criteria=u2 ~= 0
  Switch1 : Switch  Criteria=u2 ~= 0
  Switch6 : Switch  Criteria=u2 ~= 0
  TrueDurationTime5 : TrueDurationTime/TrueDurationTime  TCycle=0.02
  Unit Delay : UnitDelay  SampleTime=-1  HasFrameUpgradeWarning=on
  Unit Delay2 : UnitDelay  SampleTime=-1  HasFrameUpgradeWarning=on
  Unit Delay3 : UnitDelay  SampleTime=-1  HasFrameUpgradeWarning=on
  id1 : InportShadow
  Out1 : Outport
  wires:
  Unit Delay/1 -> Relational Operator/2
  id/1 -> Relational Operator/1, Unit Delay/1
  Switch1/1 -> Unit Delay3/1, Out1/1
  ObjType/1 -> Switch/1, Unit Delay2/1, Relational Operator1/1, Switch6/1
  Switch6/1 -> Switch/3
  TrueDurationTime5/1 -> Compare To Constant11/1
  Unit Delay2/1 -> Relational Operator1/2
  Relational Operator1/1 -> TrueDurationTime5/1
  Compare To Constant11/1 -> Switch6/2
  Unit Delay3/1 -> Switch6/3
  Constant/1 -> Switch1/1
  id1/1 -> Compare To Constant2/1
  Compare To Constant2/1 -> Switch1/2
  Switch/1 -> Switch1/3
  Relational Operator/1 -> Switch/2

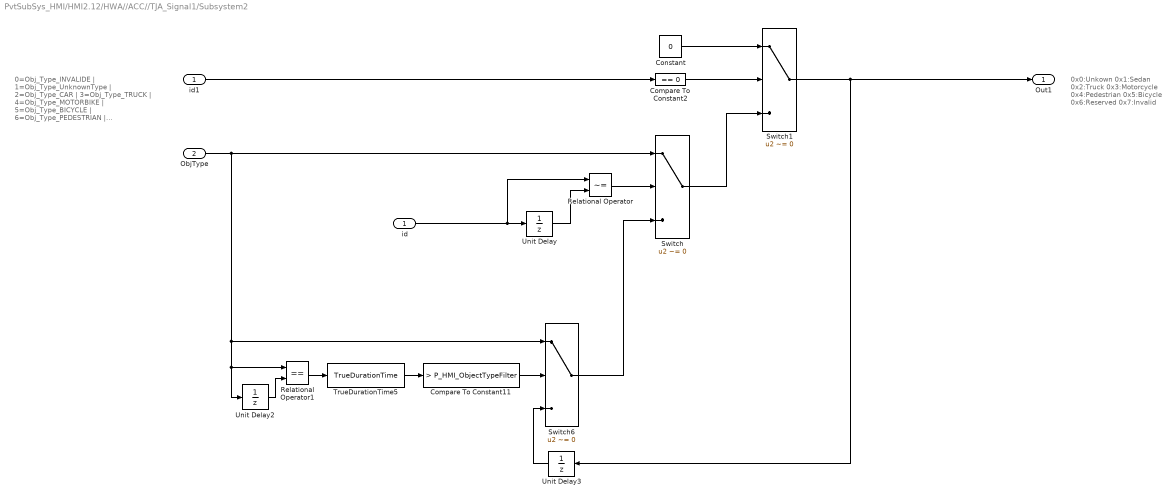
== system PvtSubSys_HMI/HMI2.12/HWA//ACC//TJA_Signal1/Subsystem2 ==
  note: 0x0:Unkown
      | 0x1:Sedan
      | 0x2:Truck
      | 0x3:Motorcycle
      | 0x4:Pedestrian
      | 0x5:Bicycle
      | 0x6:Reserved
      | 0x7:Invalid
  note: 0=Obj_Type_INVALIDE |
      | 1=Obj_Type_UnknownType |
      | 2=Obj_Type_CAR |
      | 3=Obj_Type_TRUCK |
      | 4=Obj_Type_MOTORBIKE |
      | 5=Obj_Type_BICYCLE |
      | 6=Obj_Type_PEDESTRIAN |
      | 7=Obj_Type_GENERAL_OBJECT |
      | 8=Obj_Type_ANIMAL|
  id : Inport
  ObjType : Inport  Port=2
  Compare To Constant11 : simulink/Logic and Bit Operations/Compare To Constant  relop=>  const=P_HMI_ObjectTypeFilter  OutDataTypeStr=boolean
  Compare To Constant2 : simulink/Logic and Bit Operations/Compare To Constant  relop===  const=0  OutDataTypeStr=boolean
  Constant : Constant  Value=0  OutDataTypeStr=uint8
  Relational Operator : RelationalOperator  Operator=~=  OutDataTypeStr=boolean  RndMeth=Simplest
  Relational Operator1 : RelationalOperator  Operator===  OutDataTypeStr=boolean  RndMeth=Simplest
  Switch : Switch  Criteria=u2 ~= 0
  Switch1 : Switch  Criteria=u2 ~= 0
  Switch6 : Switch  Criteria=u2 ~= 0
  TrueDurationTime5 : TrueDurationTime/TrueDurationTime  TCycle=0.02
  Unit Delay : UnitDelay  SampleTime=-1  HasFrameUpgradeWarning=on
  Unit Delay2 : UnitDelay  SampleTime=-1  HasFrameUpgradeWarning=on
  Unit Delay3 : UnitDelay  SampleTime=-1  HasFrameUpgradeWarning=on
  id1 : InportShadow
  Out1 : Outport
  wires:
  Relational Operator/1 -> Switch/2
  Switch/1 -> Switch1/3
  Compare To Constant2/1 -> Switch1/2
  id1/1 -> Compare To Constant2/1
  Constant/1 -> Switch1/1
  Unit Delay3/1 -> Switch6/3
  Compare To Constant11/1 -> Switch6/2
  Relational Operator1/1 -> TrueDurationTime5/1
  Unit Delay2/1 -> Relational Operator1/2
  TrueDurationTime5/1 -> Compare To Constant11/1
  Switch6/1 -> Switch/3
  ObjType/1 -> Switch6/1, Relational Operator1/1, Unit Delay2/1, Switch/1
  Switch1/1 -> Out1/1, Unit Delay3/1
  id/1 -> Unit Delay/1, Relational Operator/1
  Unit Delay/1 -> Relational Operator/2

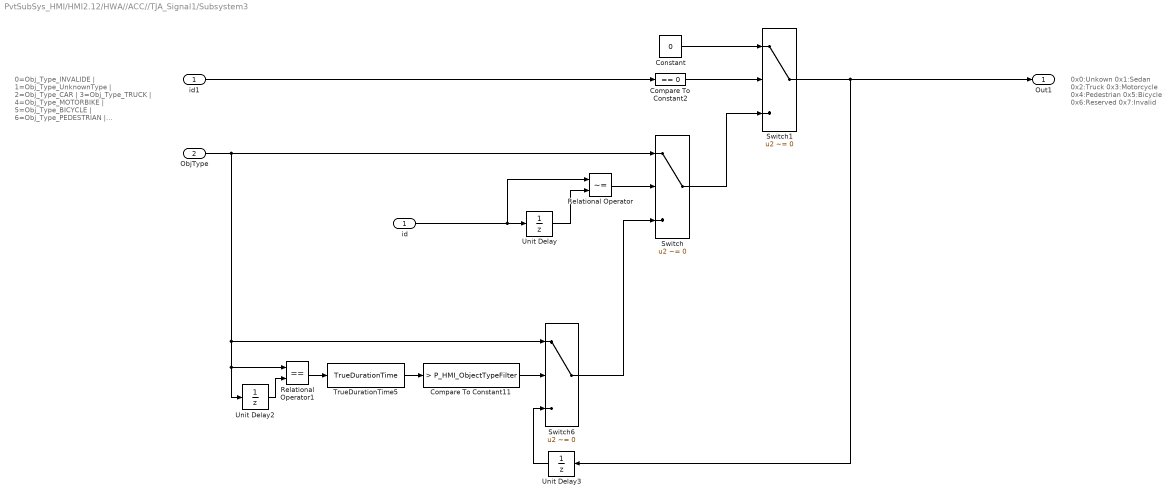
== system PvtSubSys_HMI/HMI2.12/HWA//ACC//TJA_Signal1/Subsystem3 ==
  note: 0=Obj_Type_INVALIDE |
      | 1=Obj_Type_UnknownType |
      | 2=Obj_Type_CAR |
      | 3=Obj_Type_TRUCK |
      | 4=Obj_Type_MOTORBIKE |
      | 5=Obj_Type_BICYCLE |
      | 6=Obj_Type_PEDESTRIAN |
      | 7=Obj_Type_GENERAL_OBJECT |
      | 8=Obj_Type_ANIMAL|
  note: 0x0:Unkown
      | 0x1:Sedan
      | 0x2:Truck
      | 0x3:Motorcycle
      | 0x4:Pedestrian
      | 0x5:Bicycle
      | 0x6:Reserved
      | 0x7:Invalid
  id : Inport
  ObjType : Inport  Port=2
  Compare To Constant11 : simulink/Logic and Bit Operations/Compare To Constant  relop=>  const=P_HMI_ObjectTypeFilter  OutDataTypeStr=boolean
  Compare To Constant2 : simulink/Logic and Bit Operations/Compare To Constant  relop===  const=0  OutDataTypeStr=boolean
  Constant : Constant  Value=0  OutDataTypeStr=uint8
  Relational Operator : RelationalOperator  Operator=~=  OutDataTypeStr=boolean  RndMeth=Simplest
  Relational Operator1 : RelationalOperator  Operator===  OutDataTypeStr=boolean  RndMeth=Simplest
  Switch : Switch  Criteria=u2 ~= 0
  Switch1 : Switch  Criteria=u2 ~= 0
  Switch6 : Switch  Criteria=u2 ~= 0
  TrueDurationTime5 : TrueDurationTime/TrueDurationTime  TCycle=0.02
  Unit Delay : UnitDelay  SampleTime=-1  HasFrameUpgradeWarning=on
  Unit Delay2 : UnitDelay  SampleTime=-1  HasFrameUpgradeWarning=on
  Unit Delay3 : UnitDelay  SampleTime=-1  HasFrameUpgradeWarning=on
  id1 : InportShadow
  Out1 : Outport
  wires:
  Unit Delay/1 -> Relational Operator/2
  id/1 -> Relational Operator/1, Unit Delay/1
  Switch1/1 -> Unit Delay3/1, Out1/1
  ObjType/1 -> Switch/1, Unit Delay2/1, Relational Operator1/1, Switch6/1
  Switch6/1 -> Switch/3
  TrueDurationTime5/1 -> Compare To Constant11/1
  Unit Delay2/1 -> Relational Operator1/2
  Relational Operator1/1 -> TrueDurationTime5/1
  Compare To Constant11/1 -> Switch6/2
  Unit Delay3/1 -> Switch6/3
  Constant/1 -> Switch1/1
  id1/1 -> Compare To Constant2/1
  Compare To Constant2/1 -> Switch1/2
  Switch/1 -> Switch1/3
  Relational Operator/1 -> Switch/2

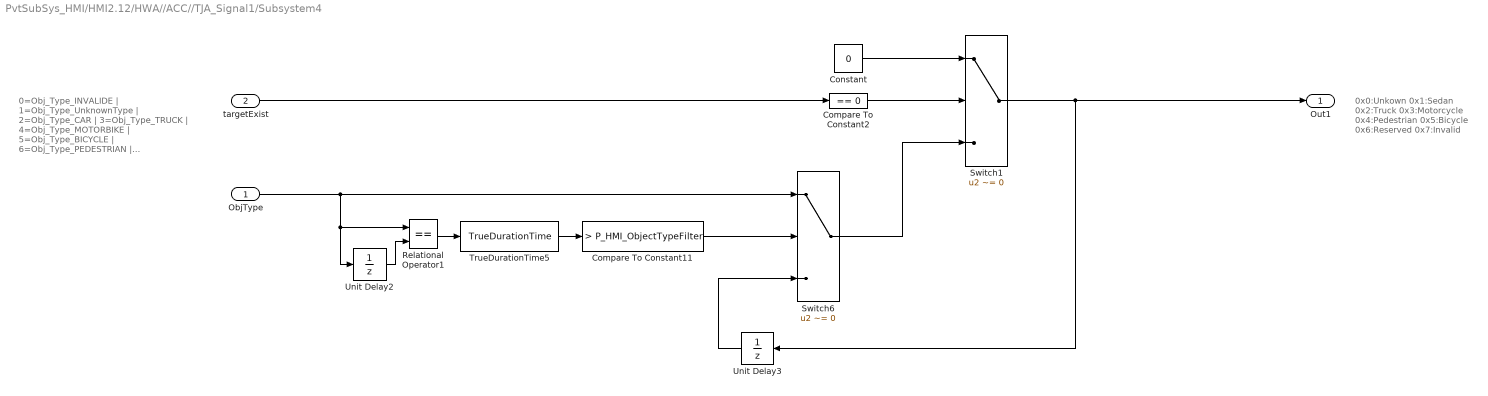
== system PvtSubSys_HMI/HMI2.12/HWA//ACC//TJA_Signal1/Subsystem4 ==
  note: 0x0:Unkown
      | 0x1:Sedan
      | 0x2:Truck
      | 0x3:Motorcycle
      | 0x4:Pedestrian
      | 0x5:Bicycle
      | 0x6:Reserved
      | 0x7:Invalid
  note: 0=Obj_Type_INVALIDE |
      | 1=Obj_Type_UnknownType |
      | 2=Obj_Type_CAR |
      | 3=Obj_Type_TRUCK |
      | 4=Obj_Type_MOTORBIKE |
      | 5=Obj_Type_BICYCLE |
      | 6=Obj_Type_PEDESTRIAN |
      | 7=Obj_Type_GENERAL_OBJECT |
      | 8=Obj_Type_ANIMAL|
  ObjType : Inport
  targetExist : Inport  Port=2
  Compare To Constant11 : simulink/Logic and Bit Operations/Compare To Constant  relop=>  const=P_HMI_ObjectTypeFilter  OutDataTypeStr=boolean
  Compare To Constant2 : simulink/Logic and Bit Operations/Compare To Constant  relop===  const=0  OutDataTypeStr=boolean
  Constant : Constant  Value=0  OutDataTypeStr=uint8
  Relational Operator1 : RelationalOperator  Operator===  OutDataTypeStr=boolean  RndMeth=Simplest
  Switch1 : Switch  Criteria=u2 ~= 0
  Switch6 : Switch  Criteria=u2 ~= 0
  TrueDurationTime5 : TrueDurationTime/TrueDurationTime  TCycle=0.02
  Unit Delay2 : UnitDelay  SampleTime=-1  HasFrameUpgradeWarning=on
  Unit Delay3 : UnitDelay  SampleTime=-1  HasFrameUpgradeWarning=on
  Out1 : Outport
  wires:
  Switch6/1 -> Switch1/3
  Compare To Constant2/1 -> Switch1/2
  targetExist/1 -> Compare To Constant2/1
  Constant/1 -> Switch1/1
  Unit Delay3/1 -> Switch6/3
  Compare To Constant11/1 -> Switch6/2
  Relational Operator1/1 -> TrueDurationTime5/1
  Unit Delay2/1 -> Relational Operator1/2
  TrueDurationTime5/1 -> Compare To Constant11/1
  ObjType/1 -> Switch6/1, Relational Operator1/1, Unit Delay2/1
  Switch1/1 -> Out1/1, Unit Delay3/1

== system PvtSubSys_HMI/HMI2.12/HWA//ACC//TJA_Signal1/Subsystem5 ==
  note: 0=Obj_Type_INVALIDE |
      | 1=Obj_Type_UnknownType |
      | 2=Obj_Type_CAR |
      | 3=Obj_Type_TRUCK |
      | 4=Obj_Type_MOTORBIKE |
      | 5=Obj_Type_BICYCLE |
      | 6=Obj_Type_PEDESTRIAN |
      | 7=Obj_Type_GENERAL_OBJECT |
      | 8=Obj_Type_ANIMAL|
  note: 0x0:Unkown
      | 0x1:Sedan
      | 0x2:Truck
      | 0x3:Motorcycle
      | 0x4:Pedestrian
      | 0x5:Bicycle
      | 0x6:Reserved
      | 0x7:Invalid
  ObjType : Inport
  targetExist : Inport  Port=2
  Compare To Constant11 : simulink/Logic and Bit Operations/Compare To Constant  relop=>  const=P_HMI_ObjectTypeFilter  OutDataTypeStr=boolean
  Compare To Constant2 : simulink/Logic and Bit Operations/Compare To Constant  relop===  const=0  OutDataTypeStr=boolean
  Constant : Constant  Value=0  OutDataTypeStr=uint8
  Relational Operator1 : RelationalOperator  Operator===  OutDataTypeStr=boolean  RndMeth=Simplest
  Switch1 : Switch  Criteria=u2 ~= 0
  Switch6 : Switch  Criteria=u2 ~= 0
  TrueDurationTime5 : TrueDurationTime/TrueDurationTime  TCycle=0.02
  Unit Delay2 : UnitDelay  SampleTime=-1  HasFrameUpgradeWarning=on
  Unit Delay3 : UnitDelay  SampleTime=-1  HasFrameUpgradeWarning=on
  Out1 : Outport
  wires:
  Switch1/1 -> Unit Delay3/1, Out1/1
  ObjType/1 -> Unit Delay2/1, Relational Operator1/1, Switch6/1
  TrueDurationTime5/1 -> Compare To Constant11/1
  Unit Delay2/1 -> Relational Operator1/2
  Relational Operator1/1 -> TrueDurationTime5/1
  Compare To Constant11/1 -> Switch6/2
  Unit Delay3/1 -> Switch6/3
  Constant/1 -> Switch1/1
  targetExist/1 -> Compare To Constant2/1
  Compare To Constant2/1 -> Switch1/2
  Switch6/1 -> Switch1/3
